simulink model "Automatic_Transmission_Controller"  (R2020b)
settings: Solver=VariableStepAuto  StartTime=0.0  StopTime=10.0  RelTol=1e-3
values from neighbouring files (symbols this model uses):
  EMAP = [-40 -44 -49 -53 -57 -61 -65 -70 -74 -78 -82;215 117 85 66 44 29 10 -2 -13 -22 -32;245 208 178 148 122 104 85 66 48 33 18;264 260 241 219 193 167 152 133 119 96 85;264 279 282 275 260 238 223 208 189 171 152;267 290 293 297 290 275 260 256 234 212 193;267 297 305 305 305 301 293 282 267 249 226;267 301 308 312 319 323 319 316 297 279 253;267 301 312 319 327 327 327 327 312 293 267;267 301 312 319  ...(+28 chars)    [Values.m]
  NE_VEC = [799.99999999999989 1200 1599.9999999999998 1999.9999999999998 2400 2800.0000000000005 3199.9999999999995 3599.9999999999995 3999.9999999999995 4400 4800]    [Values.m]
  TH_VEC = [0;20;30;40;50;60;70;80;90;100]    [Values.m]
undefined symbols (not defined in the file or in its folder): lei
settings Model: Creator=shubham sharma  LastModifiedBy=shubham sharma

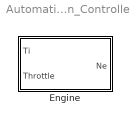
== system Automatic_Transmission_Controller ==
  Engine : Subsystem

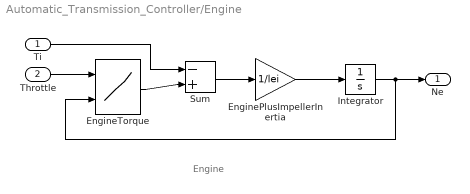
== system Automatic_Transmission_Controller/Engine ==
  note: Engine
  Ti : Inport  Unit=ft*lbf@torque
  Throttle : Inport  Port=2  Unit=%
  EnginePlusImpellerInertia : Gain  Gain=1/lei  SaturateOnIntegerOverflow=on  OutDataTypeStr=Inherit: Same as input  ParamDataTypeStr=Inherit: Same as input
  EngineTorque : Lookup_n-D  BreakpointsForDimension1=TH_VEC  BreakpointsForDimension2=NE_VEC  Table=EMAP  InputSameDT=on
      settings: InputPortMap=u0,u1
  Integrator : Integrator  InitialCondition=1000  LimitOutput=on  UpperSaturationLimit=6000  LowerSaturationLimit=600  ZeroCross=off
  Sum : Sum  Inputs=-+  InputSameDT=on  SaturateOnIntegerOverflow=on  OutDataTypeStr=Inherit: Same as first input
  Ne : Outport  Unit=rpm  VectorParamsAs1DForOutWhenUnconnected=off
  wires:
  Ti/1 -> Sum/1
  Throttle/1 -> EngineTorque/1
  Integrator/1 -> EngineTorque/2, Ne/1
  Sum/1 -> EnginePlusImpellerInertia/1
  EnginePlusImpellerInertia/1 -> Integrator/1
  EngineTorque/1 -> Sum/2
